simulink model "sistema_completo_v0"  (R2023b)
settings: Solver=VariableStepAuto  StartTime=0.0  StopTime=10.0  RelTol=1e-3
values from neighbouring files (symbols this model uses):
  alpha_Cu = 3.9e-3    (= 0.0039)    [controlador_foc_simulink.m]    (also in parametros_planta.m; params_subsistema_termico.m; sistema_completo_en_codigo.m)
  beq_nom = bm + bl_nom/r^2    (= 2.19444444444e-05)    [parametros_planta.m]    (also in params_subsistema_mecanico.m; sistema_completo_en_codigo.m)
  Cts = 0.818    [parametros_planta.m]    (also in params_subsistema_termico.m)
  Jeq_nom = Jm + Jl_nom/r^2    (= 1.97847222222e-05)    [params_subsistema_mecanico.m]    (also in sistema_completo_en_codigo.m)
  kg_eq_nom = g*kl_nom/r    (= 0.0204305208333)    [params_subsistema_mecanico.m]    (also in sistema_completo_en_codigo.m)
  L_d = 6.6e-3    (= 0.0066)    [controlador_foc_simulink.m]    (also in params_subsistema_electromagnetico.m; sistema_completo_en_codigo.m)
  L_l = 0.8e-3    (= 0.0008)    [controlador_foc_simulink.m]    (also in params_subsistema_electromagnetico.m; sistema_completo_en_codigo.m)
  L_q = 5.8e-3    (= 0.0058)    [controlador_foc_simulink.m]    (also in params_subsistema_electromagnetico.m; sistema_completo_en_codigo.m)
  lambda_m = 0.016    [controlador_foc_simulink.m]    (also in parametros_planta.m; params_subsistema_electromagnetico.m; sistema_completo_en_codigo.m)
  Pp = 3    [controlador_foc_simulink.m]    (also in parametros_planta.m; params_subsistema_electromagnetico.m; sistema_completo_en_codigo.m)
  r = 120.0    (= 120)    [controlador_foc_simulink.m]    (also in parametros_planta.m; params_subsistema_mecanico.m; sistema_completo_en_codigo.m)
  Rs_REF = 1.02    [controlador_foc_simulink.m]    (also in parametros_planta.m; params_subsistema_termico.m; sistema_completo_en_codigo.m)
  Rts_amb = 146.7    [parametros_planta.m]    (also in params_subsistema_termico.m)
  Tamb = Tamb_max    (= 40)    [parametros_planta.m]    (also in params_subsistema_termico.m; sistema_completo_en_codigo.m)
  Ts_REF = 20.0    (= 20)    [controlador_foc_simulink.m]    (also in parametros_planta.m; params_subsistema_termico.m; sistema_completo_en_codigo.m)
libraries: eeTransforms x2
settings Model: Creator=Pc  LastModifiedBy=Pc

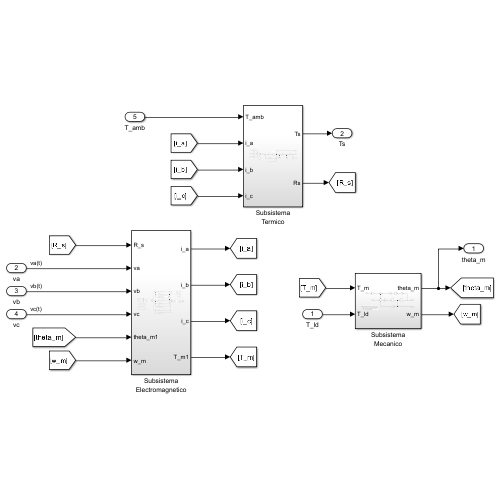
[thumbnail: Simulink's stored preview of the top-level diagram]
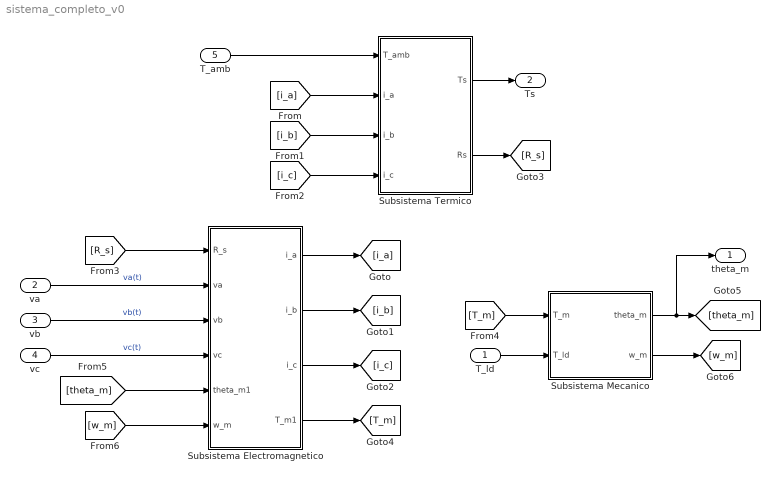
== system sistema_completo_v0 ==
  T_ld : Inport
  va : Inport  Port=2
  vb : Inport  Port=3
  vc : Inport  Port=4
  T_amb : Inport  Port=5
  Subsistema Electromagnetico : Subsystem
  Subsistema Mecanico : Subsystem
  Subsistema Termico : Subsystem
  theta_m : Outport
  Ts : Outport  Port=2
  wires:
  T_ld/1 -> Subsistema Mecanico/2(T_ld)
  Subsistema Mecanico/1(theta_m) -> theta_m/1, [theta_m]
  va/1 -> Subsistema Electromagnetico/2(va)  "va(t)"
  vb/1 -> Subsistema Electromagnetico/3(vb)  "vb(t)"
  vc/1 -> Subsistema Electromagnetico/4(vc)  "vc(t)"
  T_amb/1 -> Subsistema Termico/1(T_amb)
  Subsistema Termico/1(Ts) -> Ts/1
  Subsistema Electromagnetico/1(i_a) -> [i_a]
  [i_a] -> Subsistema Termico/2(i_a)
  Subsistema Electromagnetico/2(i_b) -> [i_b]
  Subsistema Electromagnetico/3(i_c) -> [i_c]
  [i_b] -> Subsistema Termico/3(i_b)
  [i_c] -> Subsistema Termico/4(i_c)
  Subsistema Termico/2(Rs) -> [R_s]
  [R_s] -> Subsistema Electromagnetico/1(R_s)
  Subsistema Electromagnetico/4(T_m1) -> [T_m]
  [T_m] -> Subsistema Mecanico/1(T_m)
  Subsistema Mecanico/2(w_m) -> [w_m]
  [theta_m] -> Subsistema Electromagnetico/5(theta_m1)
  [w_m] -> Subsistema Electromagnetico/6(w_m)

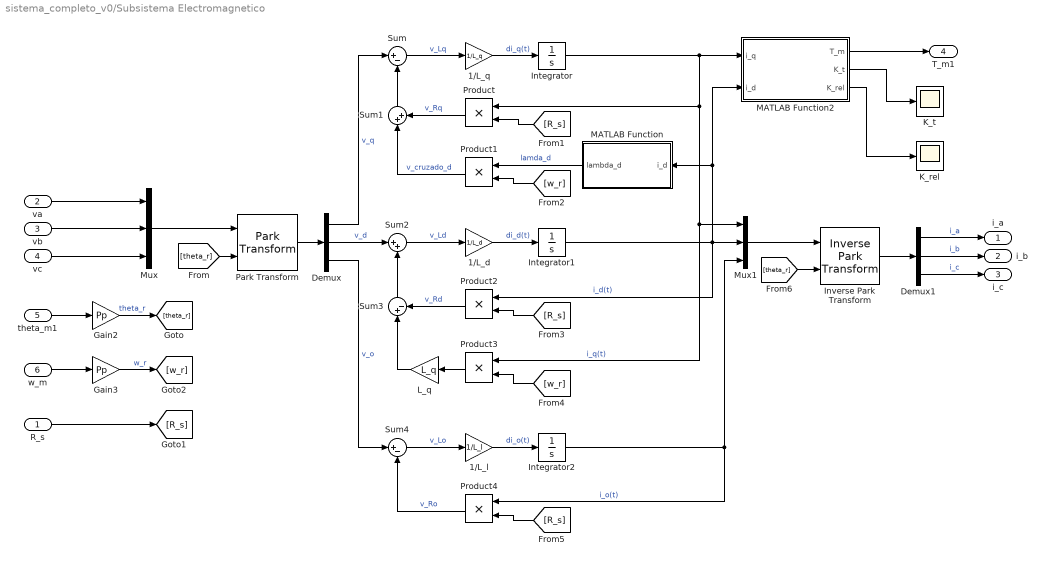
== system sistema_completo_v0/Subsistema Electromagnetico ==
  R_s : Inport
  va : Inport  Port=2
  vb : Inport  Port=3
  vc : Inport  Port=4
  theta_m1 : Inport  Port=5
  w_m : Inport  Port=6
  1/L_d : Gain  Gain=1/L_d
  1/L_l : Gain  Gain=1/L_l
  1/L_q : Gain  Gain=1/L_q
  Demux : Demux  Outputs=3
  Demux1 : Demux  Outputs=3
  Gain2 : Gain  Gain=Pp
  Gain3 : Gain  Gain=Pp
  Integrator : Integrator
  Integrator1 : Integrator
  Integrator2 : Integrator
  Inverse Park Transform : eeTransforms/Inverse Park Transform  AxisAlignment=Q-axis  PowerInvariant=off
      settings: LibrarySourceBlock=|
      | ee_sl_lib/Mathematical
      | Transforms/Inverse
      | Park Transform
  K_rel : Scope
  K_t : Scope
  L_q : Gain  Gain=L_q
  MATLAB Function : MATLAB Function  TreatAsAtomicUnit=on
  MATLAB Function2 : MATLAB Function  TreatAsAtomicUnit=on
  Mux : Mux  Inputs=3
  Mux1 : Mux  Inputs=3
  Park Transform : eeTransforms/Park Transform  AxisAlignment=Q-axis  PowerInvariant=off
      settings: LibrarySourceBlock=|
      | ee_sl_lib/Mathematical
      | Transforms/Park Transform
  Product{,1..4} (5 alike) : Product
  Sum : Sum  Inputs=|+-
  Sum1 : Sum  Inputs=|++
  Sum2 : Sum  Inputs=|++
  Sum3 : Sum  Inputs=|+-
  Sum4 : Sum  Inputs=|+-
  i_a : Outport
  i_b : Outport  Port=2
  i_c : Outport  Port=3
  T_m1 : Outport  Port=4
  wires:
  Demux1/1 -> i_a/1  "i_a"
  Product4/1 -> Sum4/2  "v_Ro"
  Park Transform/1 -> Demux/1
  1/L_l/1 -> Integrator2/1  "di_o(t)"
  Product3/1 -> L_q/1
  vb/1 -> Mux/2
  Sum3/1 -> Sum2/2
  w_m/1 -> Gain3/1
  MATLAB Function2/1(T_m) -> T_m1/1
  va/1 -> Mux/1
  [theta_r] -> Inverse Park Transform/2
  Demux/1 -> Sum/1  "v_q"
  Demux/3 -> Sum4/1  "v_o"
  Inverse Park Transform/1 -> Demux1/1
  Integrator/1 -> Product/1, Mux1/1, Product3/1, MATLAB Function2/1(i_q)  "i_q(t)"
  Demux1/3 -> i_c/1  "i_c"
  Mux/1 -> Park Transform/1
  Integrator2/1 -> Mux1/3, Product4/1  "i_o(t)"
  Gain3/1 -> [w_r]  "w_r"
  [w_r] -> Product3/2
  Sum2/1 -> 1/L_d/1  "v_Ld"
  MATLAB Function/1(lambda_d) -> Product1/1  "lamda_d"
  L_q/1 -> Sum3/1
  Integrator1/1 -> MATLAB Function/1(i_d), MATLAB Function2/2(i_d), Mux1/2, Product2/1  "i_d(t)"
  [R_s] -> Product4/2
  [theta_r] -> Park Transform/2
  Sum1/1 -> Sum/2
  [w_r] -> Product1/2
  Gain2/1 -> [theta_r]  "theta_r"
  Product1/1 -> Sum1/1  "v_cruzado_d"
  1/L_q/1 -> Integrator/1  "di_q(t)"
  [R_s] -> Product2/2
  Mux1/1 -> Inverse Park Transform/1
  R_s/1 -> [R_s]
  vc/1 -> Mux/3
  Demux1/2 -> i_b/1  "i_b"
  Demux/2 -> Sum2/1  "v_d"
  Product/1 -> Sum1/2  "v_Rq"
  theta_m1/1 -> Gain2/1
  Sum/1 -> 1/L_q/1  "v_Lq"
  MATLAB Function2/3(K_rel) -> K_rel/1
  1/L_d/1 -> Integrator1/1  "di_d(t)"
  Product2/1 -> Sum3/2  "v_Rd"
  Sum4/1 -> 1/L_l/1  "v_Lo"
  [R_s] -> Product/2
  MATLAB Function2/2(K_t) -> K_t/1

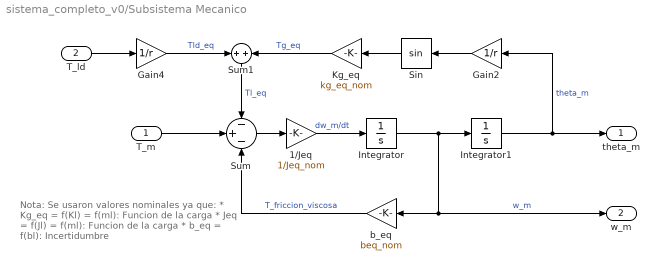
== system sistema_completo_v0/Subsistema Mecanico ==
  note: Nota: Se usaron valores nominales ya que:
      | * Kg_eq = f(Kl) = f(ml): Funcion de la carga
      | * Jeq = f(Jl) = f(ml): Funcion de la carga
      | * b_eq = f(bl): Incertidumbre
  T_m : Inport
  T_ld : Inport  Port=2
  1/Jeq : Gain  Gain=1/Jeq_nom
  Gain2 : Gain  Gain=1/r
  Gain4 : Gain  Gain=1/r
  Integrator : Integrator
  Integrator1 : Integrator
  Kg_eq : Gain  Gain=kg_eq_nom
  Sin : Trigonometry
  Sum : Sum  Inputs=-+-
  Sum1 : Sum  Inputs=+|+
  b_eq : Gain  Gain=beq_nom
  theta_m : Outport
  w_m : Outport  Port=2
  wires:
  b_eq/1 -> Sum/3  "T_friccion_viscosa"
  Integrator/1 -> w_m/1, b_eq/1, Integrator1/1  "w_m"
  Kg_eq/1 -> Sum1/2  "Tg_eq"
  Sin/1 -> Kg_eq/1
  Gain2/1 -> Sin/1
  Gain4/1 -> Sum1/1  "Tld_eq"
  Sum1/1 -> Sum/1  "Tl_eq"
  T_m/1 -> Sum/2
  Integrator1/1 -> theta_m/1, Gain2/1  "theta_m"
  T_ld/1 -> Gain4/1
  Sum/1 -> 1/Jeq/1
  1/Jeq/1 -> Integrator/1  "dw_m/dt"

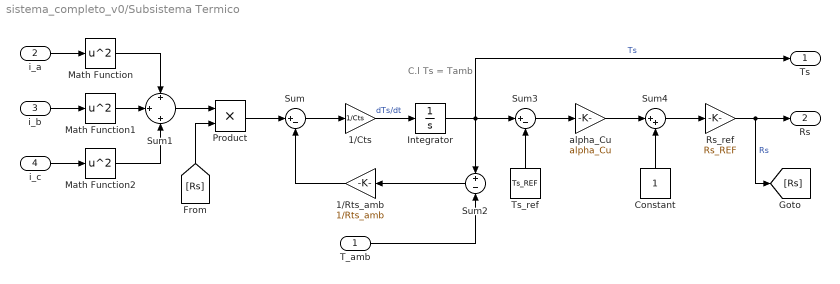
== system sistema_completo_v0/Subsistema Termico ==
  note: C.l
      | Ts = Tamb
  T_amb : Inport
  i_a : Inport  Port=2
  i_b : Inport  Port=3
  i_c : Inport  Port=4
  1/Cts : Gain  Gain=1/Cts
  1/Rts_amb : Gain  Gain=1/Rts_amb
  Constant : Constant
  Integrator : Integrator  InitialCondition=Tamb
  Math Function : Math  Operator=square
  Math Function1 : Math  Operator=square
  Math Function2 : Math  Operator=square
  Product : Product
  Rs_ref : Gain  Gain=Rs_REF
  Sum : Sum  Inputs=|+-
  Sum1 : Sum  Inputs=+|+|+
  Sum2 : Sum  Inputs=+-
  Sum3 : Sum  Inputs=|+-
  Sum4 : Sum  Inputs=|++
  Ts_ref : Constant  Value=Ts_REF
  alpha_Cu : Gain  Gain=alpha_Cu
  Ts : Outport
  Rs : Outport  Port=2
  wires:
  Integrator/1 -> Ts/1, Sum2/1, Sum3/1  "Ts"
  i_b/1 -> Math Function1/1
  Math Function1/1 -> Sum1/2
  [Rs] -> Product/2
  Rs_ref/1 -> Rs/1, [Rs]  "Rs"
  i_a/1 -> Math Function/1
  Sum1/1 -> Product/1
  Constant/1 -> Sum4/2
  Sum3/1 -> alpha_Cu/1
  Ts_ref/1 -> Sum3/2
  Product/1 -> Sum/1
  1/Rts_amb/1 -> Sum/2
  Sum2/1 -> 1/Rts_amb/1
  Math Function2/1 -> Sum1/3
  alpha_Cu/1 -> Sum4/1
  Math Function/1 -> Sum1/1
  T_amb/1 -> Sum2/2
  Sum/1 -> 1/Cts/1
  i_c/1 -> Math Function2/1
  Sum4/1 -> Rs_ref/1
  1/Cts/1 -> Integrator/1  "dTs/dt"

== matlab function sistema_completo_v0/Subsistema Electromagnetico/MATLAB Function ==
  data: i_d input; lambda_d output; lambda_m parameter; L_d parameter
function lambda_d = calcular_flujo_d(i_d, lambda_m, L_d)
    % CALCULAR_FLUJO_D Calcula el flujo magnético total concatenado en el eje directo (d).
    %
    % Entradas:
    %   i_d      : Corriente instantánea en el eje d (Señal dinámica de entrada).
    %   lambda_m : Flujo de los imanes permanentes (Parámetro estático).
    %   L_d      : Inductancia del estator en el eje d (Parámetro estático).
    %
    % Salida:
    %   lambda_d : Flujo magnético total en el eje d.

    % Cálculo: Flujo de imanes + Flujo de reacción del inducido
    lambda_d = lambda_m + L_d * i_d;
end

== matlab function sistema_completo_v0/Subsistema Electromagnetico/MATLAB Function2 ==
  data: i_q input; i_d input; T_m output; Pp parameter; lambda_m parameter; L_d parameter; L_q parameter; K_t output; K_rel output
function [T_m, K_t, K_rel] = calcular_torque(i_q, i_d, Pp, lambda_m, L_d, L_q)
    % CALCULAR_TORQUE Calcula el torque electromagnético total de la máquina PMSM
    % y sus constantes equivalentes.
    % 
    % Entradas dinámicas (Inports):
    %   i_q      : Corriente en el eje en cuadratura [A].
    %   i_d      : Corriente en el eje directo [A].
    %
    % Parámetros estáticos (Parameters):
    %   P_p      : Número de pares de polos.
    %   lambda_m : Flujo magnético de los imanes permanentes [Wb].
    %   L_d      : Inductancia del eje d [H].
    %   L_q      : Inductancia del eje q [H].
    %
    % Salidas:
    %   T_m      : Torque electromagnético generado [N.m].
    %   K_t      : Constante de torque de alineación [N.m/A].
    %   K_rel    : Constante de torque de reluctancia [N.m/A^2].

    % 1. Cálculo de las constantes 
    K_t = (3/2) * Pp * lambda_m;
    K_rel = (3/2) * Pp * (L_d - L_q);

    % 2. Cálculo del torque electromagnético total
    T_m = K_t * i_q + K_rel * i_d * i_q;
end
